simulink model "exercise_10_simscape"  (R2022b)
settings: Solver=VariableStepAuto  StartTime=0.0  StopTime=10*2*pi/w  MaxStep=(2*pi/w)*1e-4  MinStep=(2*pi/w)*1e-12  RelTol=1e-3  AbsTol=1e-3
model workspace (MAT data in the model file):
  R1 = 5
  R2 = 2
  R3 = 5
  g = 0.5
  n = 2
  w = 6.28318530718
libraries: fl_lib x12, nesl_utility x5
settings Model: Creator=stefa  LastModifiedBy=stefa
settings SolverCC: AutoScaleAbsTol=off  AlgebraicLoopSolver=TrustRegion  MaxZcPerStep=1
settings OptimizationCC: ReuseModelBlockBuffer=on
settings DebuggingCC: UnconnectedInputMsg=warning  UnconnectedOutputMsg=warning  UnconnectedLineMsg=warning  SymbolicDimsDataTypeCodeGenerationDiagnostic=none
settings ModelReferenceCC: EnableRefExpFcnMdlSchedulingChecks=on
settings SFSimCC: CustomCodeUndefinedFunction=UseInterfaceOnly
settings RTWCC: DLArmComputeVersion=19.05
settings SimscapeCC: SimscapeLogType=all  SimscapeLogSimulationStatistics=on  SimscapeLogDataHistory=10000

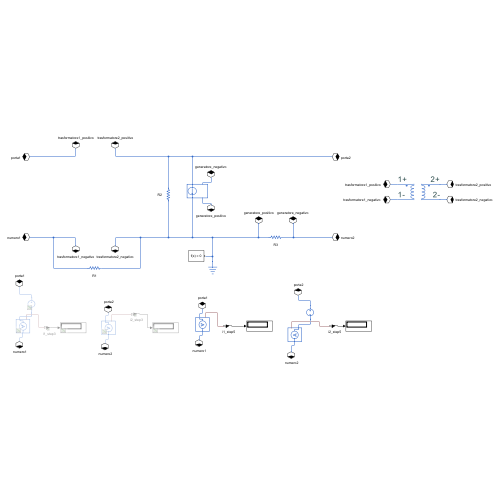
[thumbnail: Simulink's stored preview of the top-level diagram]
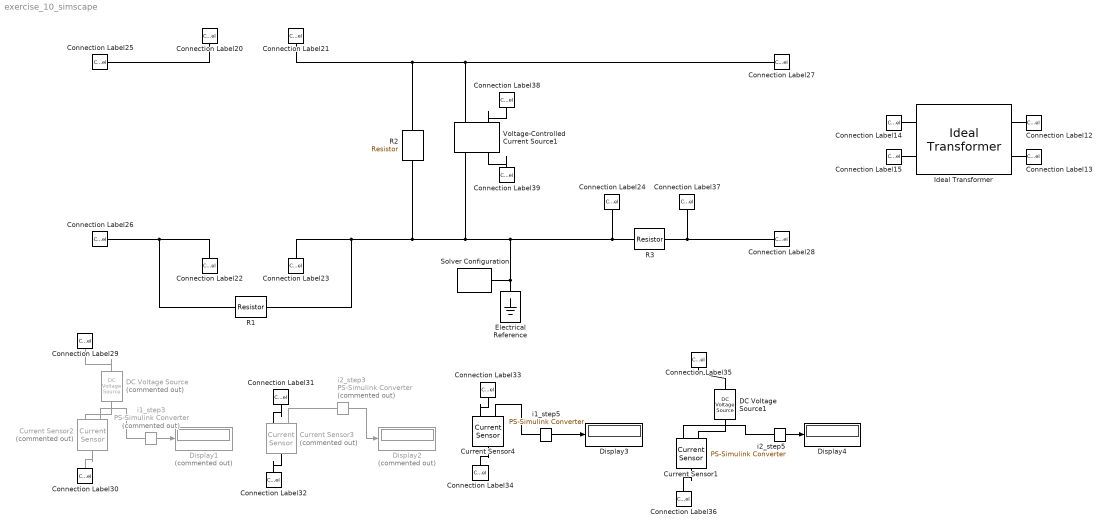
== system exercise_10_simscape ==
  Connection Label12 : ConnectionLabel  Label=trasformatore2_positivo
  Connection Label13 : ConnectionLabel  Label=trasformatore2_negativo
  Connection Label14 : ConnectionLabel  Label=trasformatore1_positivo
  Connection Label15 : ConnectionLabel  Label=trasformatore1_negativo
  Connection Label20 : ConnectionLabel  Label=trasformatore1_positivo
  Connection Label21 : ConnectionLabel  Label=trasformatore2_positivo
  Connection Label22 : ConnectionLabel  Label=trasformatore1_negativo
  Connection Label23 : ConnectionLabel  Label=trasformatore2_negativo
  Connection Label24 : ConnectionLabel  Label=generatore_positivo
  Connection Label25 : ConnectionLabel  Label=porta1
  Connection Label26 : ConnectionLabel  Label=numero1
  Connection Label27 : ConnectionLabel  Label=porta2
  Connection Label28 : ConnectionLabel  Label=numero2
  Connection Label29 : ConnectionLabel  Label=porta1
  Connection Label30 : ConnectionLabel  Label=numero1
  Connection Label31 : ConnectionLabel  Label=porta2
  Connection Label32 : ConnectionLabel  Label=numero2
  Connection Label33 : ConnectionLabel  Label=porta1
  Connection Label34 : ConnectionLabel  Label=numero1
  Connection Label35 : ConnectionLabel  Label=porta2
  Connection Label36 : ConnectionLabel  Label=numero2
  Connection Label37 : ConnectionLabel  Label=generatore_negativo
  Connection Label38 : ConnectionLabel  Label=generatore_negativo
  Connection Label39 : ConnectionLabel  Label=generatore_positivo
  Current Sensor1 : fl_lib/Electrical/Electrical Sensors/Current Sensor
  Current Sensor2 : fl_lib/Electrical/Electrical Sensors/Current Sensor  Commented=on
  Current Sensor3 : fl_lib/Electrical/Electrical Sensors/Current Sensor  Commented=on
  Current Sensor4 : fl_lib/Electrical/Electrical Sensors/Current Sensor
  DC Voltage Source : fl_lib/Electrical/Electrical Sources/DC Voltage Source  Commented=on  v0=1 V
  DC Voltage Source1 : fl_lib/Electrical/Electrical Sources/DC Voltage Source  v0=1 V
  Display1 : Display  Commented=on
  Display2 : Display  Commented=on
  Display3 : Display
  Display4 : Display
  Electrical Reference : fl_lib/Electrical/Electrical Elements/Electrical Reference
  Ideal Transformer : fl_lib/Electrical/Electrical Elements/Ideal Transformer  n=n  i1_specify=off  i1_priority=None  i1=0 A  i1_nominal_specify=off  i1_nominal_unit=A  i1_nominal_value=1  v1_specify=off  v1_priority=None  v1=0 V  v1_nominal_specify=off  v1_nominal_unit=V  v1_nominal_value=1  i2_specify=off  i2_priority=None  i2=0 A  i2_nominal_specify=off  i2_nominal_unit=A  i2_nominal_value=1  v2_specify=off  v2_priority=None  v2=0 V  v2_nominal_specify=off  v2_nominal_unit=V  v2_nominal_value=1
  R1 : fl_lib/Electrical/Electrical Elements/Resistor  R=R1 Ohm  i_specify=off  i_priority=None  i=0 A  i_nominal_specify=off  i_nominal_unit=A  i_nominal_value=1  v_specify=off  v_priority=None  v=0 V  v_nominal_specify=off  v_nominal_unit=V  v_nominal_value=1
  R2 : fl_lib/Electrical/Electrical Elements/Resistor  R=R2 Ohm  i_specify=off  i_priority=None  i=0 A  i_nominal_specify=off  i_nominal_unit=A  i_nominal_value=1  v_specify=off  v_priority=None  v=0 V  v_nominal_specify=off  v_nominal_unit=V  v_nominal_value=1
  R3 : fl_lib/Electrical/Electrical Elements/Resistor  R=R3 Ohm  i_specify=off  i_priority=None  i=0 A  i_nominal_specify=off  i_nominal_unit=A  i_nominal_value=1  v_specify=off  v_priority=None  v=0 V  v_nominal_specify=off  v_nominal_unit=V  v_nominal_value=1
  Solver Configuration : nesl_utility/Solver Configuration  PhysicalDomain=network_engine_domain  SubClassName=solver  LeftPortType=input  RightPortType=generic  Tones=[]  Harmonics=[]  SimulateNoise=off  Profile=off  UseLocalSampling=off  EnableSwitchedLinearOptims=on  FrequencyDomain=off  UseCCode=off  RelTol=0.001  AbsTol=0.001  MinStep=1e-09  ToWorkspace=off  RevertToSquareIcSolve=off  NumHomotopyIterations=100  PhasorMode=off  PhasorModeNumHarmonics=1  ConsistencySolver=NEWTON_XTOL_AFTER_FTOL  IndexReductionMethod=DerivativeReplacement  DoDC=off  ResidualTolerance=1e-09  ConsistencyTolSource=GLOBAL  ConsistencyAbsTol=0.001  ConsistencyRelTol=0.001  ConsistencyTolFactor=0.001  UseLocalSolver=off  LocalSolverChoice=NE_BACKWARD_EULER_ADVANCER  ResolveIndetEquations=on  FunctionEvalNumThread=1  LocalSolverSampleTime=0.001  DoFixedCost=off  MaxNonlinIter=3  MaxModeIter=2  ComputeImpulses=off  ImpulseIterations=2  LinearAlgebra=auto  LinearAlgebraNumThread=0  EquationFormulation=NE_TIME_EF  DelaysMemoryBudget=1024  AutomaticFiltering=on  FilteringTimeConstant=0.001  PartitionStorageMethod=AS_NEEDED  PartitionMemoryBudget=1024  PartitionMethod=ROBUST
  Voltage-Controlled Current Source1 : fl_lib/Electrical/Electrical Sources/Voltage-Controlled Current Source  K=g 1/Ohm  v1_specify=off  v1_priority=None  v1=0 V  v1_nominal_specify=off  v1_nominal_unit=V  v1_nominal_value=1  i2_specify=off  i2_priority=None  i2=0 A  i2_nominal_specify=off  i2_nominal_unit=A  i2_nominal_value=1
      settings: InternalSimscapePortConfiguration="{\"Bottom\":[],\"Left\":[{\"id\":\"p1\",\"label\":\"+\",\"type\":\"foundation.electrical.electrical\"},{\"id\":\"head\",\"label\":\"\",\"type\":\"foundation.electrical.electrical\"}],\"Right\":[{\"id\":\"n1\",\"label\":\"-\",\"type\":\"foundation.electrical.electrical\"},{\"id\":\"tail\",\"label\":\"\",\"type\":\"foundation.electrical.electrical\"}],\"Top\":[]}"
  i1_step3 : nesl_utility/PS-Simulink Converter  Commented=on  PhysicalDomain=network_engine_domain  SubClassName=ps_output  LeftPortType=input  RightPortType=output  PseudoPeriodic=off  Frequencies=[]  VectorFormat=1-D array  Unit=inherit  AffineConversion=off
  i1_step5 : nesl_utility/PS-Simulink Converter  PhysicalDomain=network_engine_domain  SubClassName=ps_output  LeftPortType=input  RightPortType=output  PseudoPeriodic=off  Frequencies=[]  VectorFormat=1-D array  Unit=inherit  AffineConversion=off
  i2_step3 : nesl_utility/PS-Simulink Converter  Commented=on  PhysicalDomain=network_engine_domain  SubClassName=ps_output  LeftPortType=input  RightPortType=output  PseudoPeriodic=off  Frequencies=[]  VectorFormat=1-D array  Unit=inherit  AffineConversion=off
  i2_step5 : nesl_utility/PS-Simulink Converter  PhysicalDomain=network_engine_domain  SubClassName=ps_output  LeftPortType=input  RightPortType=output  PseudoPeriodic=off  Frequencies=[]  VectorFormat=1-D array  Unit=inherit  AffineConversion=off
  wires:
  i1_step5/1 -> Display3/1
  i2_step5/1 -> Display4/1
  i1_step3/1 -> Display1/1
  i2_step3/1 -> Display2/1
  connections:
  Current Sensor4/LConn1 -- Connection Label34/LConn1
  Connection Label32/LConn1 -- Current Sensor3/LConn1
  Current Sensor2/RConn1 -- i1_step3/LConn1
  Current Sensor3/RConn1 -- i2_step3/LConn1
  Current Sensor1/RConn1 -- i2_step5/LConn1
  Current Sensor2/LConn1 -- Connection Label30/LConn1
  DC Voltage Source/RConn1 -- Current Sensor2/RConn2
  Current Sensor4/RConn1 -- i1_step5/LConn1
  Current Sensor1/LConn1 -- Connection Label36/LConn1
  Current Sensor4/RConn2 -- Connection Label33/LConn1
  DC Voltage Source1/LConn1 -- Connection Label35/LConn1
  Connection Label31/LConn1 -- Current Sensor3/RConn2
  DC Voltage Source/LConn1 -- Connection Label29/LConn1
  DC Voltage Source1/RConn1 -- Current Sensor1/RConn2
  Connection Label14/LConn1 -- Ideal Transformer/LConn1
  Connection Label15/LConn1 -- Ideal Transformer/LConn2
  Connection Label12/LConn1 -- Ideal Transformer/RConn1
  Connection Label13/LConn1 -- Ideal Transformer/RConn2
  Connection Label26/LConn1 -- R1/LConn1 -- Connection Label22/LConn1
  Voltage-Controlled Current Source1/RConn1 -- Connection Label38/LConn1
  Connection Label39/LConn1 -- Voltage-Controlled Current Source1/LConn1
  R2/RConn1 -- R1/RConn1 -- Connection Label23/LConn1 -- R3/LConn1 -- Connection Label24/LConn1 -- Solver Configuration/RConn1 -- Electrical Reference/LConn1 -- Voltage-Controlled Current Source1/LConn2
  R3/RConn1 -- Connection Label28/LConn1 -- Connection Label37/LConn1
  Connection Label27/LConn1 -- Voltage-Controlled Current Source1/RConn2 -- Connection Label21/LConn1 -- R2/LConn1
  Connection Label20/LConn1 -- Connection Label25/LConn1
